simulink model "calc_filter_coeff"  (Simulink 7.8)
settings: Solver=ode45  StartTime=0.0  StopTime=10.0  RelTol=1e-3
settings Model: Creator=eric  LastModifiedBy=eric

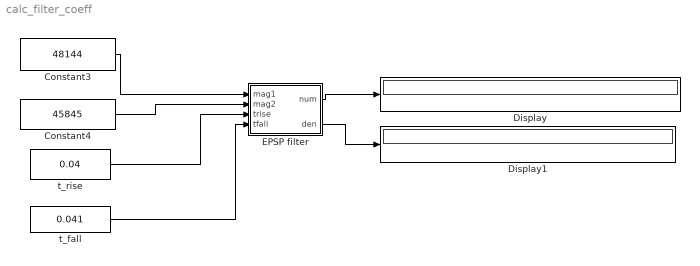
== system calc_filter_coeff ==
  Constant3 : Constant  Value=48144
  Constant4 : Constant  Value=45845
  Display : Display
      settings: Decimation=3
  Display1 : Display
      settings: Decimation=2
  EPSP filter : MATLAB Function  TreatAsAtomicUnit=on
  t_fall : Constant  Value=0.041
  t_rise : Constant  Value=0.04
  wires:
  Constant3/1 -> EPSP filter/1(mag1)
  Constant4/1 -> EPSP filter/2(mag2)
  t_rise/1 -> EPSP filter/3(trise)
  t_fall/1 -> EPSP filter/4(tfall)
  EPSP filter/1(num) -> Display/1
  EPSP filter/2(den) -> Display1/1

== matlab function EPSP filter ==
  data: num output double; den output double; mag1 input double; mag2 input double; trise input double; tfall input double
function [num, den] = fcn(mag1, mag2, trise, tfall)
%#codegen

% Shadmehr muscle model gives the h(t) of active_state
% h(t) = a*exp(-t/c) + b*exp(-t/d)
% H(s) = a/(s+c) + b/(s+d)
% This func: H(s) -> H(z) 

% a = 48144*128;
% b = 45845*128;
coder.extrinsic('tf', 'c2d', 'tfdata', 'dfilt.df2sos', 'dfilt', 'df2sos','filter'); 

a = mag1;
b = mag2;
c = 1/trise;  % tf, tr in seconds. 
d = 1/tfall;
SAMPLING_RATE = 1024; % in Hz
num = [0 (a-b) (a*d - b*c)];
den = [1 (c+d) c*d];
tf_a = tf(num, den);

tf_a_digital = c2d(tf_a, 1/SAMPLING_RATE, 'zoh');
[num den] = tfdata(tf_a_digital, 'v')
% 
% a1=den(1)
% a2=den(2)
% a3=den(3)
% b1=num(1)
% b2=num(2)
% b3=num(3)
% 
% %hd=dfilt.df2sos(b1,a1,b2,a2,b3,a3)
% bcoeff = [b1 b2 b3]
% acoeff = [a1 a2 a3]
% 
% y=[0;0]  % type definition for output
% y = filtfilt(bcoeff, acoeff,  x)
